simulink model "Controller_StepResponse"  (R2019b)
settings: Solver=VariableStepAuto  StartTime=0.0  StopTime=1000  RelTol=1e-3
undefined symbols (not defined in the file or in its folder): A, B, C, D
libraries: realtime_pacer_lib x1, simulink x1, cstblocks x1
settings Model: Creator=Presentatie  LastModifiedBy=Presentatie

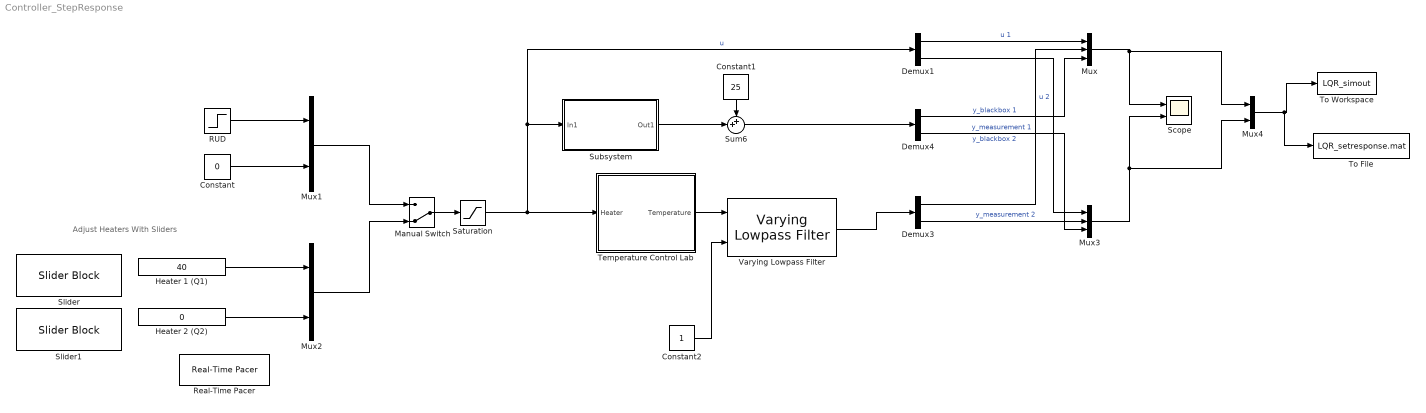
== system Controller_StepResponse ==
  note: Adjust Heaters With Sliders
  Constant : Constant  Value=0
  Constant1 : Constant  Value=25
  Constant2 : Constant
  Demux1 : Demux  Outputs=2
  Demux3 : Demux  Outputs=2
  Demux4 : Demux  Outputs=2
  Heater 1 (Q1) : Constant  Value=40
  Heater 2 (Q2) : Constant  Value=0
  Manual Switch : ManualSwitch  CurrentSetting=0
  Mux : Mux  Inputs=3
  Mux1 : Mux  Inputs=2
  Mux2 : Mux  Inputs=2
  Mux3 : Mux  Inputs=3
  Mux4 : Mux  Inputs=2
  "RUD " : Step  Time=30  After=30  SampleTime=0
  Real-Time Pacer : realtime_pacer_lib/Real-Time Pacer  simTimePerRealTime=1
  Saturation : Saturate  UpperLimit=100  LowerLimit=0
  Scope : Scope  NumInputPorts=2
  Slider : SliderBlock  TickInterval=20
  Slider1 : SliderBlock  TickInterval=20
  Subsystem : Subsystem
  Sum6 : Sum  Inputs=++|
  Temperature Control Lab : Subsystem
      mask Display: image('tclab.png');
  To File : ToFile  Filename=LQR_setresponse.mat  SaveFormat=Timeseries
  To Workspace : ToWorkspace  VariableName=LQR_simout  SaveFormat=Timeseries  SampleTime=-1
  Varying Lowpass Filter : cstblocks/Linear Parameter Varying/Varying Lowpass Filter  N=1
      settings: SourceProductName=Control System Toolbox
  wires:
  Mux/1 -> Mux4/1, Scope/1
  "RUD "/1 -> Mux1/1
  Constant/1 -> Mux1/2
  Constant1/1 -> Sum6/1
  Heater 2 (Q2)/1 -> Mux2/2
  Heater 1 (Q1)/1 -> Mux2/1
  Saturation/1 -> Demux1/1, Subsystem/1(In1), Temperature Control Lab/1(Heater)  "u"
  Mux3/1 -> Mux4/2, Scope/2
  Mux4/1 -> To Workspace/1, To File/1
  Sum6/1 -> Demux4/1
  Subsystem/1(Out1) -> Sum6/2
  Demux1/1 -> Mux/1  "u 1"
  Demux1/2 -> Mux3/1  "u 2"
  Demux4/1 -> Mux/3  "y_blackbox 1"
  Demux3/1 -> Mux/2  "y_measurement 1"
  Demux3/2 -> Mux3/2  "y_measurement 2"
  Demux4/2 -> Mux3/3  "y_blackbox 2"
  Mux2/1 -> Manual Switch/2
  Mux1/1 -> Manual Switch/1
  Manual Switch/1 -> Saturation/1
  Temperature Control Lab/1(Temperature) -> Varying Lowpass Filter/1
  Varying Lowpass Filter/1 -> Demux3/1
  Constant2/1 -> Varying Lowpass Filter/2

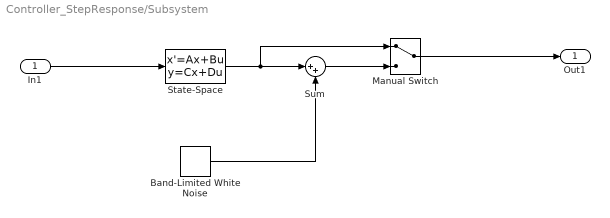
== system Controller_StepResponse/Subsystem ==
  In1 : Inport
  Band-Limited White Noise : simulink/Sources/Band-Limited White Noise  Cov=[0.1]  Ts=0.1  seed=[23341]
  Manual Switch : ManualSwitch
  State-Space : StateSpace  A=A  B=B  C=C  D=D  InitialCondition=0
  Sum : Sum  Inputs=|++
  Out1 : Outport
  wires:
  In1/1 -> State-Space/1
  Band-Limited White Noise/1 -> Sum/2
  State-Space/1 -> Manual Switch/1, Sum/1
  Sum/1 -> Manual Switch/2
  Manual Switch/1 -> Out1/1

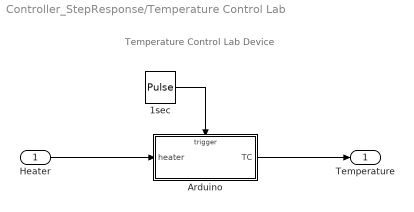
== system Controller_StepResponse/Temperature Control Lab ==
  note: Temperature Control Lab Device
  Heater : Inport
  1sec : DiscretePulseGenerator  PulseType=Time based  Period=1  PulseWidth=50
  Arduino : Subsystem  TreatAsAtomicUnit=on
  Temperature : Outport  VectorParamsAs1DForOutWhenUnconnected=off
  wires:
  1sec/1 -> Arduino/Trigger
  Arduino/1(TC) -> Temperature/1
  Heater/1 -> Arduino/1(heater)

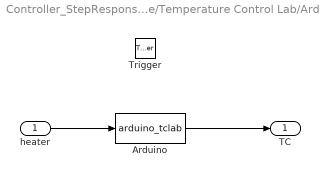
== system Controller_StepResponse/Temperature Control Lab/Arduino ==
  heater : Inport  LatchByDelayingOutsideSignal=on
  Trigger : TriggerPort  VariantControl=Variant
  Arduino : MATLABFcn  MATLABFcn=arduino_tclab
  TC : Outport  InitialOutput=[23 23]  VectorParamsAs1DForOutWhenUnconnected=off
  wires:
  heater/1 -> Arduino/1
  Arduino/1 -> TC/1
